simulink model "elevateur_NL_BO_Devoir_1"  (R2023a)
settings: Solver=ode45  StartTime=0.0  StopTime=15  RelTol=1e-3  EnableMultiTasking=on
undefined symbols (not defined in the file): Bt, current_d, current_T, J, Ka, Kt1, Kt3
settings Model: Creator=Administrateur  LastModifiedBy=abmahi
settings SolverCC: AlgebraicLoopSolver=TrustRegion
settings DataIOCC: LimitDataPoints=on  SaveFormat=Array  SignalLoggingSaveFormat=ModelDataLogs  ReturnWorkspaceOutputs=off
settings OptimizationCC: ExpressionDepthLimit=2147483647  InitFltsAndDblsToZero=on  LifeSpan=inf
settings DebuggingCC: UnderspecifiedInitializationDetection=Classic  MergeDetectMultiDrivingBlocksExec=none  SolverPrmCheckMsg=warning  FcnCallInpInsideContextMsg=warning  UnconnectedInputMsg=warning  UnconnectedOutputMsg=warning  UnconnectedLineMsg=warning  AllowSymbolicDim=off  StateNameClashWarn=warning  SFUnexpectedBacktrackingDiag=warning  SFNoUnconditionalDefaultTransitionDiag=warning  SFExecutionAtInitializationDiag=none  ArithmeticOperatorsInVariantConditions=warning
settings HardwareCC: ProdBitPerPointer=32  ProdBitPerSizeT=32  ProdBitPerPtrDiffT=32  ProdLargestAtomicFloat=None  ProdIntDivRoundTo=Undefined  ProdEndianess=Unspecified  ProdWordSize=32  ProdHWDeviceType=32-bit Generic
settings ModelReferenceCC: EnableRefExpFcnMdlSchedulingChecks=on  PropagateSignalLabelsOutOfModel=off
settings SFSimCC: SimUseLocalCustomCode=off  CustomCodeUndefinedFunction=UseInterfaceOnly
settings RTWCC: RTWUseLocalCustomCode=off
settings CodeAppCC: StateflowObjectComments=on
settings GRTTargetCC: TargetLangStandard=C89/C90 (ANSI)  CombineOutputUpdateFcns=off  GRTInterface=on
settings ConfigComp: CovMetricSettings=dw  CovSaveCumulativeToWorkspaceVar=on  CovSaveSingleToWorkspaceVar=on  CovExternalEMLEnable=off

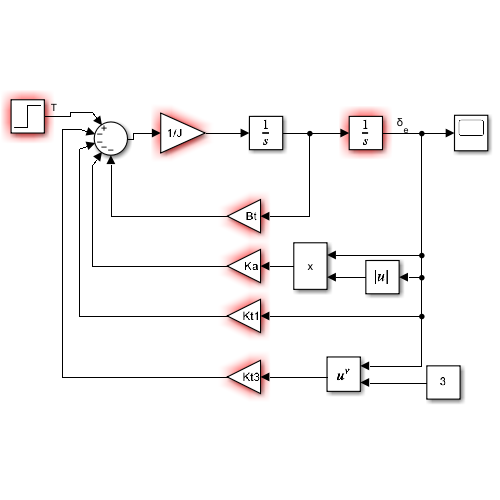
[thumbnail: Simulink's stored preview of the top-level diagram]
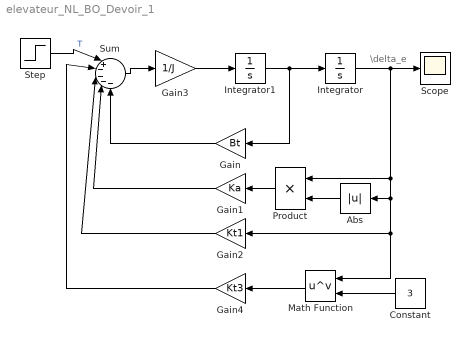
== system elevateur_NL_BO_Devoir_1 ==
  note: \delta_e
  Abs : Abs  SaturateOnIntegerOverflow=off
  Constant : Constant  Value=3
  Gain : Gain  Gain=Bt
  Gain1 : Gain  Gain=Ka
  Gain2 : Gain  Gain=Kt1
  Gain3 : Gain  Gain=1/J
  Gain4 : Gain  Gain=Kt3
  Integrator : Integrator  InitialCondition=current_d
  Integrator1 : Integrator
  Math Function : Math  Operator=pow
  Product : Product
  Scope : Scope
  Step : Step  Time=0  After=current_T  SampleTime=0
  Sum : Sum  Inputs=|+----
  wires:
  Integrator1/1 -> Integrator/1, Gain/1
  Sum/1 -> Gain3/1
  Gain/1 -> Sum/5
  Gain1/1 -> Sum/4
  Gain3/1 -> Integrator1/1
  Product/1 -> Gain1/1
  Integrator/1 -> Scope/1, Math Function/1, Gain2/1, Abs/1, Product/1
  Abs/1 -> Product/2
  Step/1 -> Sum/1  "T"
  Constant/1 -> Math Function/2
  Gain2/1 -> Sum/3
  Gain4/1 -> Sum/2
  Math Function/1 -> Gain4/1
